simulink model "df_simulation"  (R2018b)
settings: Solver=FixedStepAuto  StartTime=0.0  StopTime=100  FixedStep=0.01  RelTol=1e-3
values from neighbouring files (symbols this model uses):
  B = [-C1,  O1, I3, Z3, Z3, Z3 ... (first row only)    [set_df_simulation.m]
  invBa = inv(Ba)    [set_df_simulation.m]
  invBd = inv(Bd)    [set_df_simulation.m]
  invBe = eye(3)    [set_df_simulation.m]
libraries: simulink x23, cstblocks x13
settings Model: Creator=sho  LastModifiedBy=sho

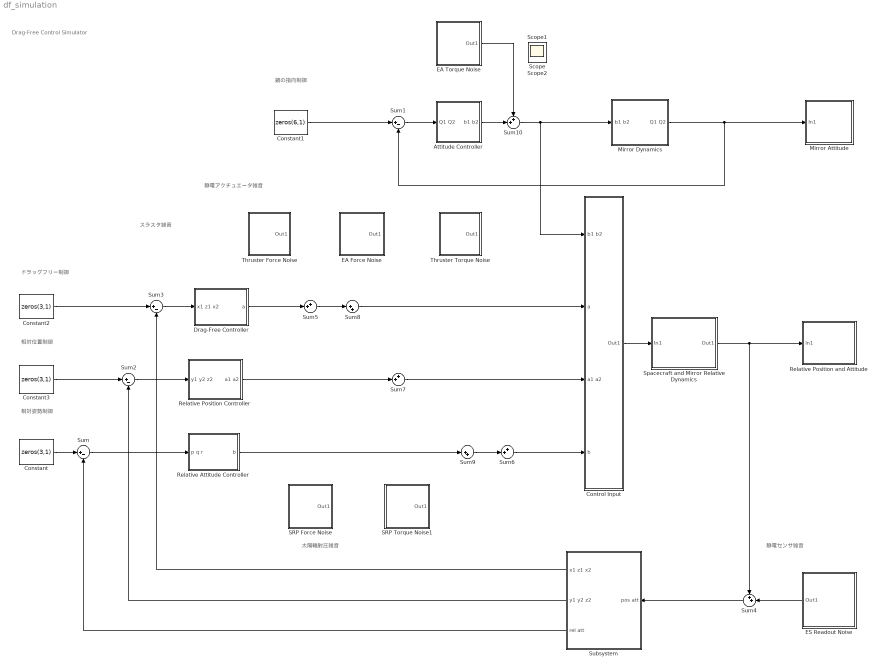
== system df_simulation ==
  note: Drag-Free Control Simulator
  note: 相対位置制御
  note: ドラッグフリー制御
  note: 相対姿勢制御
  note: 鏡の指向制御
  note: 静電アクチュエータ雑音
  note: スラスタ雑音
  note: 静電センサ雑音
  note: 太陽輻射圧雑音
  Attitude Controller : Subsystem
  Constant : Constant  Value=zeros(3,1)
  Constant1 : Constant  Value=zeros(6,1)
  Constant2 : Constant  Value=zeros(3,1)
  Constant3 : Constant  Value=zeros(3,1)
  Control Input : Subsystem
  Drag-Free Controller : Subsystem
  EA Force Noise : Subsystem
  EA Torque Noise : Subsystem
  ES Readout Noise : Subsystem
  Mirror Attitude : Subsystem
  "Mirror Dynamics " : Subsystem
  Relative Attitude Controller : Subsystem
  Relative Position Controller : Subsystem
  Relative Position and Attitude : Subsystem
  SRP Force Noise : Subsystem
  SRP Torque Noise1 : Subsystem
  Spacecraft and Mirror Relative Dynamics : Subsystem
  Subsystem : Subsystem
  Sum{,1..3} (4 alike) : Sum  Inputs=|+-
  Sum{4..7,10} (5 alike) : Sum  Inputs=++|
  Sum8 : Sum  Inputs=|++
  Sum9 : Sum  Inputs=|++
  Thruster Force Noise : Subsystem
  Thruster Torque Noise : Subsystem
  Scope : Scope
  Scope1 : Scope
  Scope2 : Scope
  wires:
  Constant/1 -> Sum/1
  Sum/1 -> Relative Attitude Controller/1(p q r)
  Constant1/1 -> Sum1/1
  Sum1/1 -> Attitude Controller/1(Q1 Q2)
  "Mirror Dynamics "/1(Q1 Q2) -> Sum1/2, Mirror Attitude/1(In1)
  Control Input/1(Out1) -> Spacecraft and Mirror Relative Dynamics/1(In1)
  Spacecraft and Mirror Relative Dynamics/1(Out1) -> Relative Position and Attitude/1(In1), Sum4/1
  Constant2/1 -> Sum3/1
  Constant3/1 -> Sum2/1
  Sum3/1 -> Drag-Free Controller/1(x1 z1 x2)
  Sum2/1 -> Relative Position Controller/1(y1 y2 z2)
  Sum4/1 -> Subsystem/1(pos att)
  Subsystem/1(x1 z1 x2) -> Sum3/2
  Subsystem/2(y1 y2 z2) -> Sum2/2
  Subsystem/3(rel att) -> Sum/2
  Drag-Free Controller/1(a) -> Sum5/2
  Sum6/1 -> Control Input/4(b)
  Relative Position Controller/1(a1 a2) -> Sum7/2
  Sum7/1 -> Control Input/3(a1 a2)
  Sum5/1 -> Sum8/1
  Sum8/1 -> Control Input/2(a)
  Sum9/1 -> Sum6/2
  Relative Attitude Controller/1(b) -> Sum9/1
  Attitude Controller/1(b1 b2) -> Sum10/2
  Sum10/1 -> Control Input/1(b1 b2), "Mirror Dynamics "/1(b1 b2)
  EA Torque Noise/1(Out1) -> Sum10/1
  ES Readout Noise/1(Out1) -> Sum4/2

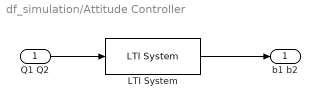
== system df_simulation/Attitude Controller ==
  Q1 Q2 : Inport
  LTI System : cstblocks/LTI System  sys=Kaa  IC=[]
  b1 b2 : Outport
  wires:
  Q1 Q2/1 -> LTI System/1
  LTI System/1 -> b1 b2/1

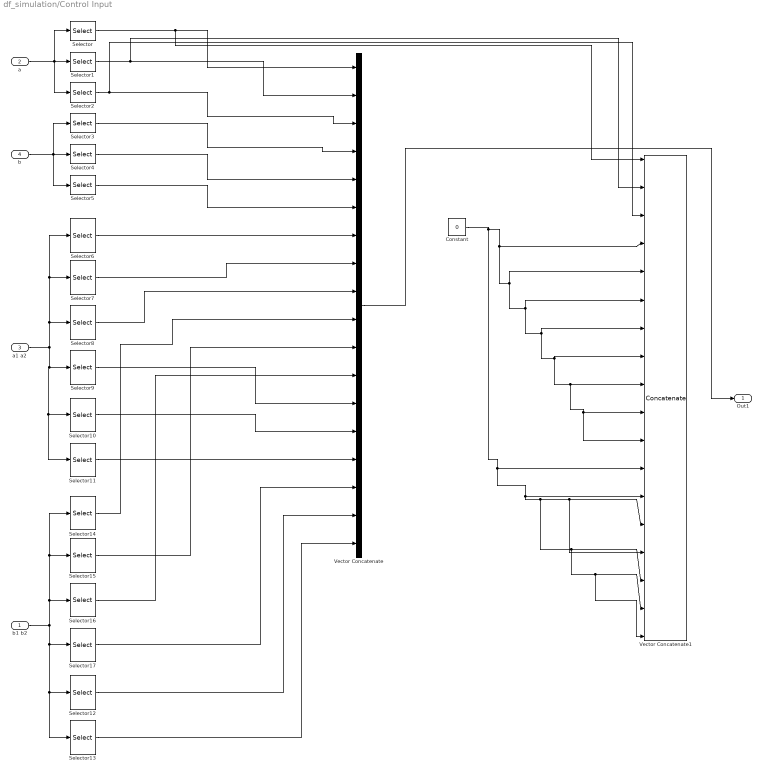
== system df_simulation/Control Input ==
  b1 b2 : Inport
  a : Inport  Port=2
  a1 a2 : Inport  Port=3
  b : Inport  Port=4
  Constant : Constant  Value=0
  Selector : Selector  InputPortWidth=3  IndexOptions=Index vector (dialog)  Indices=1  OutputSizes=1
  Selector1 : Selector  InputPortWidth=3  IndexOptions=Index vector (dialog)  Indices=2  OutputSizes=1
  Selector10 : Selector  InputPortWidth=6  IndexOptions=Index vector (dialog)  Indices=5  OutputSizes=1
  Selector11 : Selector  InputPortWidth=6  IndexOptions=Index vector (dialog)  Indices=6  OutputSizes=1
  Selector12 : Selector  InputPortWidth=6  IndexOptions=Index vector (dialog)  Indices=5  OutputSizes=1
  Selector13 : Selector  InputPortWidth=6  IndexOptions=Index vector (dialog)  Indices=6  OutputSizes=1
  Selector14 : Selector  InputPortWidth=6  IndexOptions=Index vector (dialog)  Indices=1  OutputSizes=1
  Selector15 : Selector  InputPortWidth=6  IndexOptions=Index vector (dialog)  Indices=2  OutputSizes=1
  Selector16 : Selector  InputPortWidth=6  IndexOptions=Index vector (dialog)  Indices=3  OutputSizes=1
  Selector17 : Selector  InputPortWidth=6  IndexOptions=Index vector (dialog)  Indices=4  OutputSizes=1
  Selector2 : Selector  InputPortWidth=3  IndexOptions=Index vector (dialog)  Indices=3  OutputSizes=1
  Selector3 : Selector  InputPortWidth=3  IndexOptions=Index vector (dialog)  Indices=1  OutputSizes=1
  Selector4 : Selector  InputPortWidth=3  IndexOptions=Index vector (dialog)  Indices=2  OutputSizes=1
  Selector5 : Selector  InputPortWidth=3  IndexOptions=Index vector (dialog)  Indices=3  OutputSizes=1
  Selector6 : Selector  InputPortWidth=6  IndexOptions=Index vector (dialog)  Indices=1  OutputSizes=1
  Selector7 : Selector  InputPortWidth=6  IndexOptions=Index vector (dialog)  Indices=2  OutputSizes=1
  Selector8 : Selector  InputPortWidth=6  IndexOptions=Index vector (dialog)  Indices=3  OutputSizes=1
  Selector9 : Selector  InputPortWidth=6  IndexOptions=Index vector (dialog)  Indices=4  OutputSizes=1
  Vector Concatenate : Concatenate  NumInputs=18
  Vector Concatenate1 : Concatenate  NumInputs=18
  Out1 : Outport
  wires:
  a/1 -> Selector/1, Selector2/1, Selector1/1
  Selector/1 -> Vector Concatenate1/1, Vector Concatenate/1
  Selector1/1 -> Vector Concatenate1/2, Vector Concatenate/2
  Selector2/1 -> Vector Concatenate1/3, Vector Concatenate/3
  b/1 -> Selector3/1, Selector5/1, Selector4/1
  Selector3/1 -> Vector Concatenate/4
  Selector4/1 -> Vector Concatenate/5
  Selector5/1 -> Vector Concatenate/6
  a1 a2/1 -> Selector11/1, Selector10/1, Selector9/1, Selector8/1, Selector7/1, Selector6/1
  Selector7/1 -> Vector Concatenate/8
  Selector8/1 -> Vector Concatenate/9
  b1 b2/1 -> Selector17/1, Selector12/1, Selector13/1, Selector16/1, Selector15/1, Selector14/1
  Selector17/1 -> Vector Concatenate/16
  Selector12/1 -> Vector Concatenate/17
  Selector13/1 -> Vector Concatenate/18
  Selector14/1 -> Vector Concatenate/10
  Selector15/1 -> Vector Concatenate/11
  Selector16/1 -> Vector Concatenate/12
  Selector9/1 -> Vector Concatenate/13
  Selector10/1 -> Vector Concatenate/14
  Selector11/1 -> Vector Concatenate/15
  Selector6/1 -> Vector Concatenate/7
  Constant/1 -> Vector Concatenate1/18, Vector Concatenate1/17, Vector Concatenate1/16, Vector Concatenate1/15, Vector Concatenate1/14, Vector Concatenate1/13, Vector Concatenate1/12, Vector Concatenate1/11, Vector Concatenate1/10, Vector Concatenate1/9, Vector Concatenate1/8, Vector Concatenate1/7, Vector Concatenate1/6, Vector Concatenate1/5, Vector Concatenate1/4
  Vector Concatenate/1 -> Out1/1

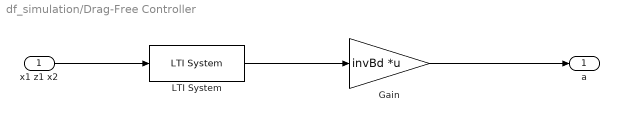
== system df_simulation/Drag-Free Controller ==
  x1 z1 x2 : Inport
  Gain : Gain  Gain=invBd  Multiplication=Matrix(K*u) (u vector)
  LTI System : cstblocks/LTI System  sys=Kd  IC=[]
  a : Outport
  wires:
  LTI System/1 -> Gain/1
  Gain/1 -> a/1
  x1 z1 x2/1 -> LTI System/1

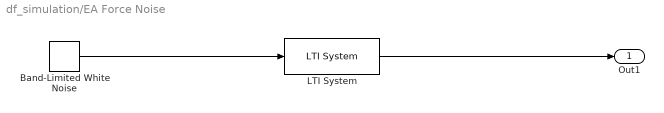
== system df_simulation/EA Force Noise ==
  Band-Limited White Noise : simulink/Sources/Band-Limited White Noise  Cov=ones(6,1)  Ts=0.01  seed=[23341]  VectorParams1D=off
  LTI System : cstblocks/LTI System  sys=Wespp  IC=[]
  Out1 : Outport
  wires:
  Band-Limited White Noise/1 -> LTI System/1
  LTI System/1 -> Out1/1

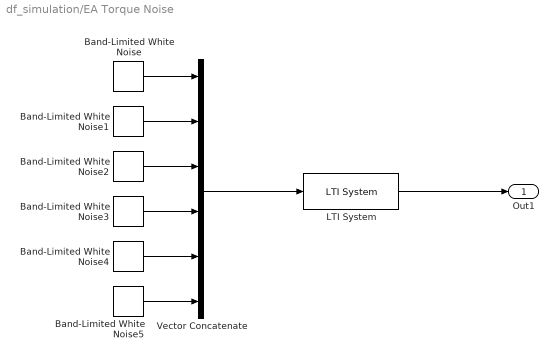
== system df_simulation/EA Torque Noise ==
  Band-Limited White Noise : simulink/Sources/Band-Limited White Noise  Cov=1  Ts=0.01  seed=[23341]
  Band-Limited White Noise1 : simulink/Sources/Band-Limited White Noise  Cov=1  Ts=0.01  seed=[23346]
  Band-Limited White Noise2 : simulink/Sources/Band-Limited White Noise  Cov=1  Ts=0.01  seed=[23342]
  Band-Limited White Noise3 : simulink/Sources/Band-Limited White Noise  Cov=1  Ts=0.01  seed=[23343]
  Band-Limited White Noise4 : simulink/Sources/Band-Limited White Noise  Cov=1  Ts=0.01  seed=[23344]
  Band-Limited White Noise5 : simulink/Sources/Band-Limited White Noise  Cov=1  Ts=0.01  seed=[23345]
  LTI System : cstblocks/LTI System  sys=Wesaa  IC=[]
  Vector Concatenate : Concatenate  NumInputs=6
  Out1 : Outport
  wires:
  LTI System/1 -> Out1/1
  Vector Concatenate/1 -> LTI System/1
  Band-Limited White Noise/1 -> Vector Concatenate/1
  Band-Limited White Noise2/1 -> Vector Concatenate/3
  Band-Limited White Noise3/1 -> Vector Concatenate/4
  Band-Limited White Noise4/1 -> Vector Concatenate/5
  Band-Limited White Noise5/1 -> Vector Concatenate/6
  Band-Limited White Noise1/1 -> Vector Concatenate/2

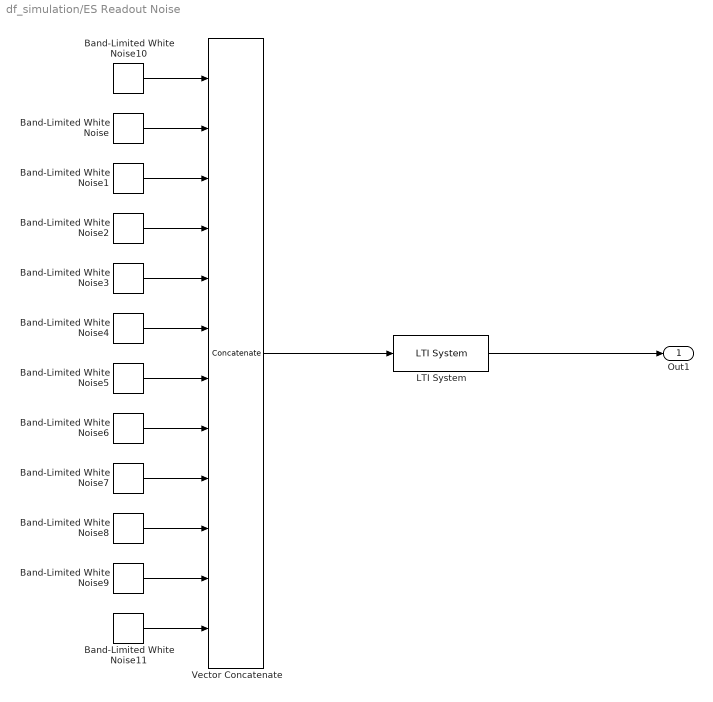
== system df_simulation/ES Readout Noise ==
  Band-Limited White Noise{,1..11} (12 alike) : simulink/Sources/Band-Limited White Noise  Cov=1  Ts=0.01  seed=[23341]
  LTI System : cstblocks/LTI System  sys=Wisq  IC=[]
  Vector Concatenate : Concatenate  NumInputs=12
  Out1 : Outport
  wires:
  Band-Limited White Noise10/1 -> Vector Concatenate/1
  Band-Limited White Noise/1 -> Vector Concatenate/2
  Band-Limited White Noise1/1 -> Vector Concatenate/3
  Band-Limited White Noise2/1 -> Vector Concatenate/4
  Band-Limited White Noise3/1 -> Vector Concatenate/5
  Band-Limited White Noise11/1 -> Vector Concatenate/12
  Band-Limited White Noise9/1 -> Vector Concatenate/11
  Band-Limited White Noise8/1 -> Vector Concatenate/10
  Band-Limited White Noise7/1 -> Vector Concatenate/9
  Band-Limited White Noise6/1 -> Vector Concatenate/8
  Band-Limited White Noise5/1 -> Vector Concatenate/7
  Band-Limited White Noise4/1 -> Vector Concatenate/6
  Vector Concatenate/1 -> LTI System/1
  LTI System/1 -> Out1/1

== system df_simulation/Mirror Attitude ==
  In1 : Inport
  To Workspace : ToWorkspace  VariableName=log_att  SaveFormat=Timeseries  SampleTime=-1
  wires:
  In1/1 -> To Workspace/1

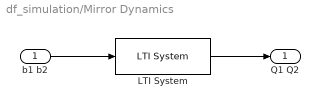
== system df_simulation/Mirror Dynamics  ==
  b1 b2 : Inport
  LTI System : cstblocks/LTI System  sys=Pm  IC=[]
  Q1 Q2 : Outport
  wires:
  b1 b2/1 -> LTI System/1
  LTI System/1 -> Q1 Q2/1

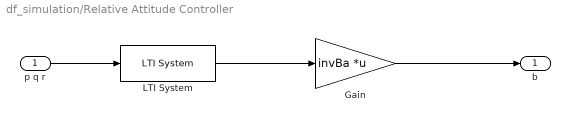
== system df_simulation/Relative Attitude Controller ==
  p q r : Inport
  Gain : Gain  Gain=invBa  Multiplication=Matrix(K*u) (u vector)
  LTI System : cstblocks/LTI System  sys=Kra  IC=[]
  b : Outport
  wires:
  p q r/1 -> LTI System/1
  LTI System/1 -> Gain/1
  Gain/1 -> b/1

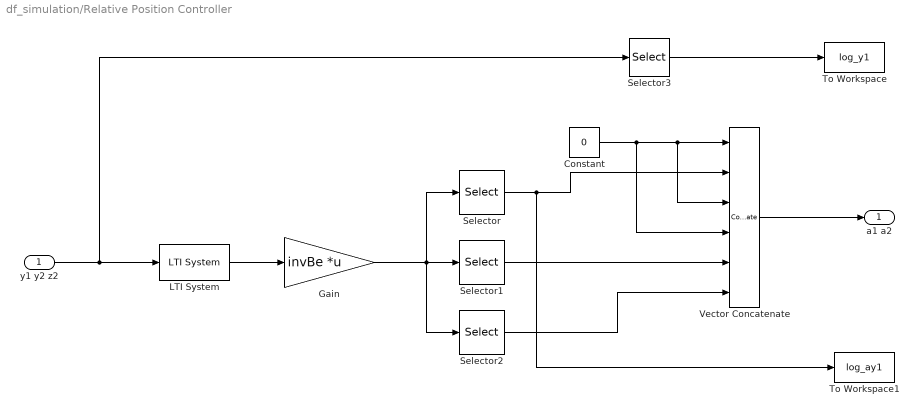
== system df_simulation/Relative Position Controller ==
  y1 y2 z2 : Inport
  Constant : Constant  Value=0
  Gain : Gain  Gain=invBe  Multiplication=Matrix(K*u) (u vector)
  LTI System : cstblocks/LTI System  sys=Krp  IC=[]
  Selector : Selector  InputPortWidth=3  IndexOptions=Index vector (dialog)  Indices=1  OutputSizes=1
  Selector1 : Selector  InputPortWidth=3  IndexOptions=Index vector (dialog)  Indices=2  OutputSizes=1
  Selector2 : Selector  InputPortWidth=3  IndexOptions=Index vector (dialog)  Indices=3  OutputSizes=1
  Selector3 : Selector  InputPortWidth=3  IndexOptions=Index vector (dialog)  Indices=1  OutputSizes=1
  To Workspace : ToWorkspace  VariableName=log_y1  SaveFormat=Timeseries  SampleTime=-1
  To Workspace1 : ToWorkspace  VariableName=log_ay1  SaveFormat=Timeseries  SampleTime=-1
  Vector Concatenate : Concatenate  NumInputs=6
  a1 a2 : Outport
  wires:
  y1 y2 z2/1 -> Selector3/1, LTI System/1
  Vector Concatenate/1 -> a1 a2/1
  Constant/1 -> Vector Concatenate/4, Vector Concatenate/3, Vector Concatenate/1
  LTI System/1 -> Gain/1
  Gain/1 -> Selector2/1, Selector/1, Selector1/1
  Selector/1 -> To Workspace1/1, Vector Concatenate/2
  Selector1/1 -> Vector Concatenate/5
  Selector2/1 -> Vector Concatenate/6
  Selector3/1 -> To Workspace/1

== system df_simulation/Relative Position and Attitude ==
  In1 : Inport
  To Workspace : ToWorkspace  VariableName=log_rel  SaveFormat=Timeseries  SampleTime=-1
  wires:
  In1/1 -> To Workspace/1

== system df_simulation/SRP Force Noise ==
  Band-Limited White Noise : simulink/Sources/Band-Limited White Noise  Cov=ones(3,1)  Ts=0.01  seed=[23341]  VectorParams1D=off
  LTI System : cstblocks/LTI System  sys=Wsrpp  IC=[]
  Out1 : Outport
  wires:
  Band-Limited White Noise/1 -> LTI System/1
  LTI System/1 -> Out1/1

== system df_simulation/SRP Torque Noise1 ==
  Band-Limited White Noise : simulink/Sources/Band-Limited White Noise  Cov=ones(3,1)  Ts=0.01  seed=[23341]  VectorParams1D=off
  LTI System : cstblocks/LTI System  sys=Wsrpa  IC=[]
  Out1 : Outport
  wires:
  Band-Limited White Noise/1 -> LTI System/1
  LTI System/1 -> Out1/1

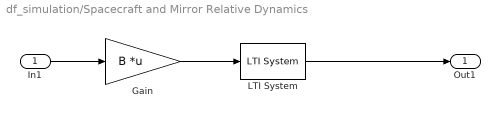
== system df_simulation/Spacecraft and Mirror Relative Dynamics ==
  In1 : Inport
  Gain : Gain  Gain=B  Multiplication=Matrix(K*u) (u vector)
  LTI System : cstblocks/LTI System  sys=Pq  IC=[]
  Out1 : Outport
  wires:
  In1/1 -> Gain/1
  Gain/1 -> LTI System/1
  LTI System/1 -> Out1/1

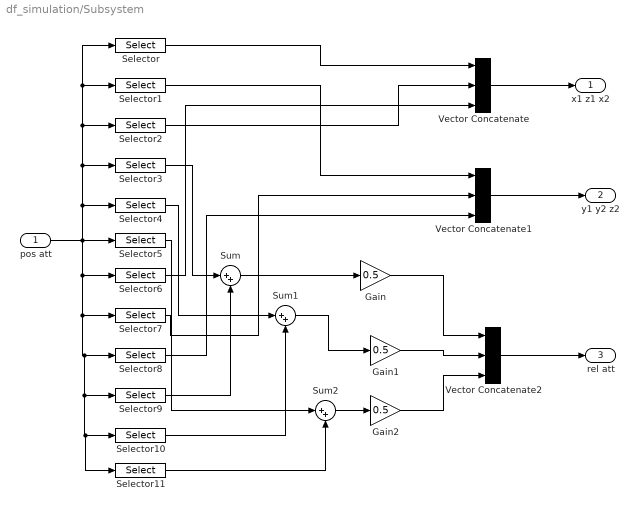
== system df_simulation/Subsystem ==
  pos att : Inport
  Gain : Gain  Gain=0.5
  Gain1 : Gain  Gain=0.5
  Gain2 : Gain  Gain=0.5
  Selector : Selector  InputPortWidth=12  IndexOptions=Index vector (dialog)  Indices=1  OutputSizes=1
  Selector1 : Selector  InputPortWidth=12  IndexOptions=Index vector (dialog)  Indices=2  OutputSizes=1
  Selector10 : Selector  InputPortWidth=12  IndexOptions=Index vector (dialog)  Indices=11  OutputSizes=1
  Selector11 : Selector  InputPortWidth=12  IndexOptions=Index vector (dialog)  Indices=12  OutputSizes=1
  Selector2 : Selector  InputPortWidth=12  IndexOptions=Index vector (dialog)  Indices=3  OutputSizes=1
  Selector3 : Selector  InputPortWidth=12  IndexOptions=Index vector (dialog)  Indices=4  OutputSizes=1
  Selector4 : Selector  InputPortWidth=12  IndexOptions=Index vector (dialog)  Indices=5  OutputSizes=1
  Selector5 : Selector  InputPortWidth=12  IndexOptions=Index vector (dialog)  Indices=6  OutputSizes=1
  Selector6 : Selector  InputPortWidth=12  IndexOptions=Index vector (dialog)  Indices=7  OutputSizes=1
  Selector7 : Selector  InputPortWidth=12  IndexOptions=Index vector (dialog)  Indices=8  OutputSizes=1
  Selector8 : Selector  InputPortWidth=12  IndexOptions=Index vector (dialog)  Indices=9  OutputSizes=1
  Selector9 : Selector  InputPortWidth=12  IndexOptions=Index vector (dialog)  Indices=10  OutputSizes=1
  Sum : Sum  Inputs=|++
  Sum1 : Sum  Inputs=|++
  Sum2 : Sum  Inputs=|++
  Vector Concatenate : Concatenate  NumInputs=3
  Vector Concatenate1 : Concatenate  NumInputs=3
  Vector Concatenate2 : Concatenate  NumInputs=3
  x1 z1 x2 : Outport
  y1 y2 z2 : Outport  Port=2
  rel att : Outport  Port=3
  wires:
  Vector Concatenate2/1 -> rel att/1
  Vector Concatenate1/1 -> y1 y2 z2/1
  Vector Concatenate/1 -> x1 z1 x2/1
  pos att/1 -> Selector11/1, Selector10/1, Selector9/1, Selector8/1, Selector7/1, Selector6/1, Selector5/1, Selector4/1, Selector3/1, Selector2/1, Selector1/1, Selector/1
  Sum/1 -> Gain/1
  Gain/1 -> Vector Concatenate2/1
  Sum1/1 -> Gain1/1
  Gain1/1 -> Vector Concatenate2/2
  Sum2/1 -> Gain2/1
  Gain2/1 -> Vector Concatenate2/3
  Selector/1 -> Vector Concatenate/1
  Selector1/1 -> Vector Concatenate1/1
  Selector2/1 -> Vector Concatenate/2
  Selector3/1 -> Sum/1
  Selector4/1 -> Sum1/1
  Selector5/1 -> Sum2/1
  Selector6/1 -> Vector Concatenate/3
  Selector7/1 -> Vector Concatenate1/2
  Selector8/1 -> Vector Concatenate1/3
  Selector9/1 -> Sum/2
  Selector10/1 -> Sum1/2
  Selector11/1 -> Sum2/2

== system df_simulation/Thruster Force Noise ==
  Band-Limited White Noise : simulink/Sources/Band-Limited White Noise  Cov=ones(3,1)  Ts=0.01  seed=[23341]  VectorParams1D=off
  LTI System : cstblocks/LTI System  sys=Wthrp  IC=[]
  Out1 : Outport
  wires:
  Band-Limited White Noise/1 -> LTI System/1
  LTI System/1 -> Out1/1

== system df_simulation/Thruster Torque Noise ==
  Band-Limited White Noise : simulink/Sources/Band-Limited White Noise  Cov=ones(3,1)  Ts=0.01  seed=[23341]  VectorParams1D=off
  LTI System : cstblocks/LTI System  sys=Wthra  IC=[]
  Out1 : Outport
  wires:
  Band-Limited White Noise/1 -> LTI System/1
  LTI System/1 -> Out1/1
